simulink model "smc_mass_1d"  (R2015a)
settings: Solver=ode3  StartTime=0.0  StopTime=tsim  FixedStep=ts  RelTol=1e-3
values from neighbouring files (symbols this model uses):
  B = 0.2    [run_simu.m]
  M = 1    [run_simu.m]
settings Model: Creator=auralius  LastModifiedBy=auralius
settings SolverCC: AlgebraicLoopSolver=LineSearch
settings SimMechanicsCC: VisDuringSimulation=on

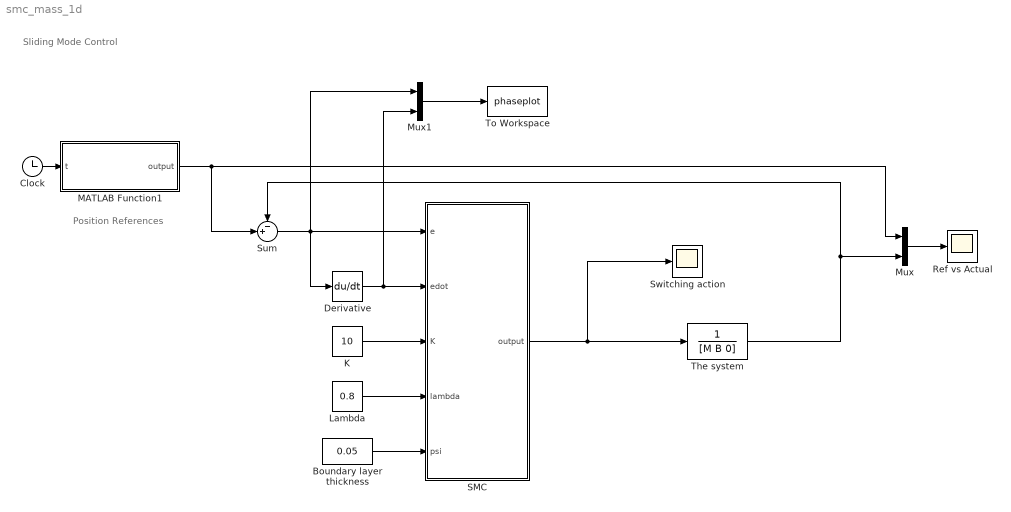
== system smc_mass_1d ==
  note: Sliding Mode Control
  note: Position References
  Boundary layer thickness : Constant  Value=0.05
  Clock : Clock
  Derivative : Derivative
  K : Constant  Value=10
  Lambda : Constant  Value=0.8
  MATLAB Function1 : MATLAB Function  TreatAsAtomicUnit=on
  Mux : Mux  Inputs=2
  Mux1 : Mux  Inputs=2
  Ref vs Actual : Scope
  SMC : MATLAB Function  TreatAsAtomicUnit=on
  Sum : Sum  Inputs=-+|
  Switching action : Scope
  The system : TransferFcn  Denominator=[M B 0]
  To Workspace : ToWorkspace  VariableName=phaseplot  SampleTime=-1
  wires:
  The system/1 -> Sum/1, Mux/2
  Derivative/1 -> Mux1/2, SMC/2(edot)
  Sum/1 -> Mux1/1, SMC/1(e), Derivative/1
  Lambda/1 -> SMC/4(lambda)
  K/1 -> SMC/3(K)
  Boundary layer thickness/1 -> SMC/5(psi)
  Mux/1 -> Ref vs Actual/1
  SMC/1(output) -> The system/1, Switching action/1
  MATLAB Function1/1(output) -> Mux/1, Sum/2
  Clock/1 -> MATLAB Function1/1(t)
  Mux1/1 -> To Workspace/1

== matlab function smc_mass_1d/SMC ==
  data: e input; output output; edot input; K input; lambda input; psi input
function output = smc(e, edot, K, lambda, psi)
%#codegen

    s = lambda * e + edot;
        
    if (abs(s) > psi)    
        sat_s = sign(s);
    else
        sat_s = s/psi;
    end
    
    output = -(edot - K * sat_s);

end

== matlab function smc_mass_1d/MATLAB Function1 ==
  data: t input; output output
function output = generate_input(t)
%#codegen

    output = -pi/2+52.5/180*pi*(1-cos(1.26*t));
end
